simulink model "exitstate_violate_conditionstate"  (R2024a)
settings: Solver=FixedStepDiscrete  StartTime=0.0  StopTime=10.0  RelTol=1e-3
settings Model: Creator=VICTUS  LastModifiedBy=VICTUS

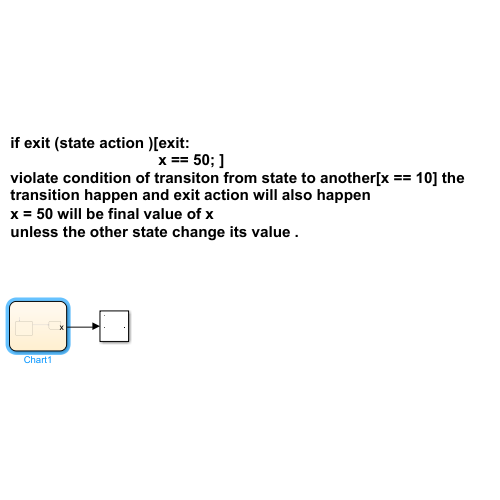
[thumbnail: Simulink's stored preview of the top-level diagram]
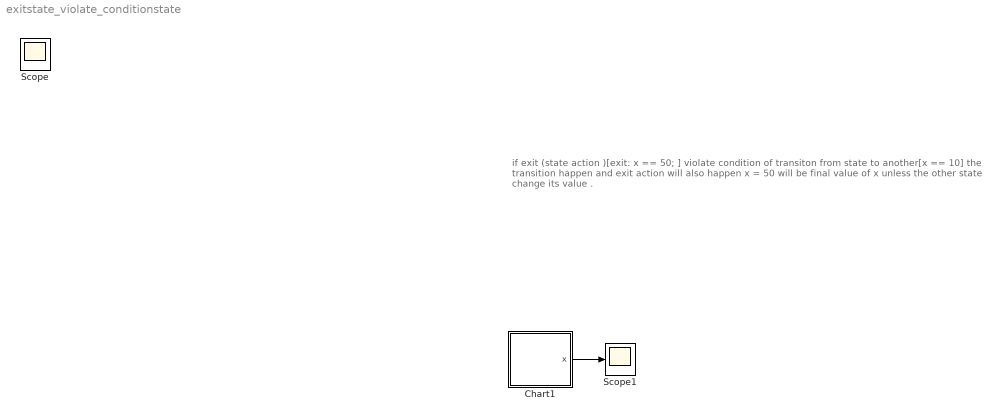
== system exitstate_violate_conditionstate ==
  note: if exit (state action )[exit:
      | x == 50; ]
      | violate condition of transiton from state to another[x == 10] the transition happen and exit action will also happen
      | x = 50 will be final value of x
      | unless the other state change its value .
  Chart1 : Stateflow chart  TreatAsAtomicUnit=on
  Scope1 : Scope
  Scope : Scope
  wires:
  Chart1/1(x) -> Scope1/1

== stateflow chart exitstate_violate_conditionstate/Chart1 ==
  state a
    en:
    x = 0;
    du:
    x = x+1;
    exit:
    x = 50;
  state b
    en:
    x = 1;
  (default) -> a
  a -> b : [x == 10]{x = 5}
  data: x output
